simulink model "gm_uz_pmsm_model_6LUT_pd_vnl"  (R2023b)
settings: Solver=FixedStepAuto  StartTime=0.0  StopTime=0.05  RelTol=1e-3
PreLoadFcn:
  | uz_pmsm_model_init_parameter
PostLoadFcn:
  | % Import the data from Excel for a lookup table
  | FluxMapData = readtable('C:\Users\Philipp\ultrazohm\ultrazohm_sw\ip_cores\uz_pmsm_model\FluxMapData_2023-05-26_13-07-57.csv');
  | % Row indices for lookup table
  | d_current_in_d_axis = FluxMapData(8:27,1:end);
  | % Column indices for lookup table
  | q_current_in_d_axis = FluxMapData(29:48,1:end);
  | % Output values for lookup table
  | d_Flux_d_axis = FluxMapData(50:69,1:end);
undefined symbols (not defined in the file or in its folder): ad1, ad2, ad3, ad4, ad5, ad6, aq1, aq2, aq3, aq4, aq5, aq6, d_current_d_Flux, d_current_q_Flux, entkopplung_dynamic, entkopplung_linear, entkopplung_static, Fid1_Giq1, Fid2_Giq2, Flux_d, Flux_q, friction_coefficient, inertia, Ki_Bo_d, Ki_Bo_q, Kp_Bo_d, Kp_Bo_q, L_d, L_q, Ldq, parameter_nachfuerung, polepair, praediktion_entkopplung_nonlinear, psi_pm, q_current_d_Flux, q_current_q_Flux, R_1, simulate_mechanical, simulate_nonlinear_modell, simulate_open_loop, static_friction_torque, tau_sum, ts, ts_regler
libraries: hdlmdlgenlib x19, simulink x2, slpidlib x2
(part 4 of 4)

== system gm_uz_pmsm_model_6LUT_pd_vnl/uz_pmsm_model_6LUT/Product41 ==
  In1 : Inport
  In2 : Inport  Port=2
  Product41 : Product  Inputs=**  OutDataTypeStr=double  SampleTime=1e-08
  Product41_pd1 : Delay  DelayLength=6
  Out1 : Outport
  wires:
  Product41_pd1/1 -> Out1/1
  Product41/1 -> Product41_pd1/1
  In2/1 -> Product41/2
  In1/1 -> Product41/1

== system gm_uz_pmsm_model_6LUT_pd_vnl/uz_pmsm_model_6LUT/Product42 ==
  In1 : Inport
  In2 : Inport  Port=2
  Product42 : Product  Inputs=**  OutDataTypeStr=double  SampleTime=1e-08
  Product42_pd1 : Delay  DelayLength=6
  Out1 : Outport
  wires:
  Product42_pd1/1 -> Out1/1
  Product42/1 -> Product42_pd1/1
  In2/1 -> Product42/2
  In1/1 -> Product42/1

== system gm_uz_pmsm_model_6LUT_pd_vnl/uz_pmsm_model_6LUT/Product43 ==
  In1 : Inport
  In2 : Inport  Port=2
  Product43 : Product  Inputs=**  OutDataTypeStr=double  SampleTime=1e-08
  Product43_pd1 : Delay  DelayLength=6
  Out1 : Outport
  wires:
  Product43_pd1/1 -> Out1/1
  Product43/1 -> Product43_pd1/1
  In2/1 -> Product43/2
  In1/1 -> Product43/1

== system gm_uz_pmsm_model_6LUT_pd_vnl/uz_pmsm_model_6LUT/Product5 ==
  In1 : Inport
  In2 : Inport  Port=2
  Product5 : Product  Inputs=**  OutDataTypeStr=double  SampleTime=1e-08
  Product5_pd1 : Delay  DelayLength=6
  Out1 : Outport
  wires:
  Product5_pd1/1 -> Out1/1
  Product5/1 -> Product5_pd1/1
  In2/1 -> Product5/2
  In1/1 -> Product5/1

== system gm_uz_pmsm_model_6LUT_pd_vnl/uz_pmsm_model_6LUT/Product51 ==
  In1 : Inport
  In2 : Inport  Port=2
  Product51 : Product  Inputs=**  OutDataTypeStr=double  SampleTime=1e-08
  Product51_pd1 : Delay  DelayLength=6
  Out1 : Outport
  wires:
  Product51_pd1/1 -> Out1/1
  Product51/1 -> Product51_pd1/1
  In2/1 -> Product51/2
  In1/1 -> Product51/1

== system gm_uz_pmsm_model_6LUT_pd_vnl/uz_pmsm_model_6LUT/Product52 ==
  In1 : Inport
  In2 : Inport  Port=2
  Product52 : Product  Inputs=**  OutDataTypeStr=double  SampleTime=1e-08
  Product52_pd1 : Delay  DelayLength=6
  Out1 : Outport
  wires:
  Product52_pd1/1 -> Out1/1
  Product52/1 -> Product52_pd1/1
  In2/1 -> Product52/2
  In1/1 -> Product52/1

== system gm_uz_pmsm_model_6LUT_pd_vnl/uz_pmsm_model_6LUT/Product6 ==
  In1 : Inport
  In2 : Inport  Port=2
  Product6 : Product  Inputs=**  OutDataTypeStr=double  SampleTime=1e-08
  Product6_pd1 : Delay  DelayLength=6
  Out1 : Outport
  wires:
  Product6_pd1/1 -> Out1/1
  Product6/1 -> Product6_pd1/1
  In2/1 -> Product6/2
  In1/1 -> Product6/1

== system gm_uz_pmsm_model_6LUT_pd_vnl/uz_pmsm_model_6LUT/Product61 ==
  In1 : Inport
  In2 : Inport  Port=2
  Product61 : Product  Inputs=**  OutDataTypeStr=double  SampleTime=1e-08
  Product61_pd1 : Delay  DelayLength=6
  Out1 : Outport
  wires:
  Product61_pd1/1 -> Out1/1
  Product61/1 -> Product61_pd1/1
  In2/1 -> Product61/2
  In1/1 -> Product61/1

== system gm_uz_pmsm_model_6LUT_pd_vnl/uz_pmsm_model_6LUT/Product7 ==
  In1 : Inport
  In2 : Inport  Port=2
  Product7 : Product  Inputs=**  OutDataTypeStr=double  SampleTime=1e-08
  Product7_pd1 : Delay  DelayLength=6
  Out1 : Outport
  wires:
  Product7_pd1/1 -> Out1/1
  Product7/1 -> Product7_pd1/1
  In2/1 -> Product7/2
  In1/1 -> Product7/1

== system gm_uz_pmsm_model_6LUT_pd_vnl/uz_pmsm_model_6LUT/Product71 ==
  In1 : Inport
  In2 : Inport  Port=2
  Product71 : Product  Inputs=**  OutDataTypeStr=double  SampleTime=1e-08
  Product71_pd1 : Delay  DelayLength=6
  Out1 : Outport
  wires:
  Product71_pd1/1 -> Out1/1
  Product71/1 -> Product71_pd1/1
  In2/1 -> Product71/2
  In1/1 -> Product71/1

== system gm_uz_pmsm_model_6LUT_pd_vnl/uz_pmsm_model_6LUT/Product7_to_gain ==
  In1 : Inport
  Product7_to_gain : Gain  Gain=double(0.5)
  Product7_to_gain_pd1 : Delay  DelayLength=3
  Out1 : Outport
  wires:
  Product7_to_gain_pd1/1 -> Out1/1
  Product7_to_gain/1 -> Product7_to_gain_pd1/1
  In1/1 -> Product7_to_gain/1

== system gm_uz_pmsm_model_6LUT_pd_vnl/uz_pmsm_model_6LUT/Product8 ==
  In1 : Inport
  In2 : Inport  Port=2
  Product8 : Product  Inputs=**  OutDataTypeStr=double  SampleTime=1e-08
  Product8_pd1 : Delay  DelayLength=6
  Out1 : Outport
  wires:
  Product8_pd1/1 -> Out1/1
  Product8/1 -> Product8_pd1/1
  In2/1 -> Product8/2
  In1/1 -> Product8/1

== system gm_uz_pmsm_model_6LUT_pd_vnl/uz_pmsm_model_6LUT/Product81 ==
  In1 : Inport
  In2 : Inport  Port=2
  Product81 : Product  Inputs=*/  OutDataTypeStr=double  SampleTime=1e-08
  Product81_pd1 : Delay  DelayLength=31
  Out1 : Outport
  wires:
  Product81_pd1/1 -> Out1/1
  Product81/1 -> Product81_pd1/1
  In2/1 -> Product81/2
  In1/1 -> Product81/1

== system gm_uz_pmsm_model_6LUT_pd_vnl/uz_pmsm_model_6LUT/Product9 ==
  In1 : Inport
  In2 : Inport  Port=2
  Product9 : Product  Inputs=**  OutDataTypeStr=double  SampleTime=1e-08
  Product9_pd1 : Delay  DelayLength=6
  Out1 : Outport
  wires:
  Product9_pd1/1 -> Out1/1
  Product9/1 -> Product9_pd1/1
  In2/1 -> Product9/2
  In1/1 -> Product9/1

== system gm_uz_pmsm_model_6LUT_pd_vnl/uz_pmsm_model_6LUT/Product91 ==
  In1 : Inport
  In2 : Inport  Port=2
  Product91 : Product  Inputs=**  OutDataTypeStr=double  SampleTime=1e-08
  Product91_pd1 : Delay  DelayLength=6
  Out1 : Outport
  wires:
  Product91_pd1/1 -> Out1/1
  Product91/1 -> Product91_pd1/1
  In2/1 -> Product91/2
  In1/1 -> Product91/1

== system gm_uz_pmsm_model_6LUT_pd_vnl/uz_pmsm_model_6LUT/Product92 ==
  In1 : Inport
  In2 : Inport  Port=2
  Product92 : Product  Inputs=**  OutDataTypeStr=double  SampleTime=1e-08
  Product92_pd1 : Delay  DelayLength=6
  Out1 : Outport
  wires:
  Product92_pd1/1 -> Out1/1
  Product92/1 -> Product92_pd1/1
  In2/1 -> Product92/2
  In1/1 -> Product92/1

== system gm_uz_pmsm_model_6LUT_pd_vnl/uz_pmsm_model_6LUT/Product93 ==
  In1 : Inport
  In2 : Inport  Port=2
  Product93 : Product  Inputs=**  OutDataTypeStr=double  SampleTime=1e-08
  Product93_pd1 : Delay  DelayLength=6
  Out1 : Outport
  wires:
  Product93_pd1/1 -> Out1/1
  Product93/1 -> Product93_pd1/1
  In2/1 -> Product93/2
  In1/1 -> Product93/1

== system gm_uz_pmsm_model_6LUT_pd_vnl/uz_pmsm_model_6LUT/Product94 ==
  In1 : Inport
  In2 : Inport  Port=2
  Product94 : Product  Inputs=*/  OutDataTypeStr=double  SampleTime=1e-08
  Product94_pd1 : Delay  DelayLength=31
  Out1 : Outport
  wires:
  Product94_pd1/1 -> Out1/1
  Product94/1 -> Product94_pd1/1
  In2/1 -> Product94/2
  In1/1 -> Product94/1

== system gm_uz_pmsm_model_6LUT_pd_vnl/uz_pmsm_model_6LUT/Sign1 ==
  In1 : Inport
  Sign1 : Signum  SampleTime=1e-08
  Out1 : Outport
  wires:
  Sign1/1 -> Out1/1
  In1/1 -> Sign1/1

== system gm_uz_pmsm_model_6LUT_pd_vnl/uz_pmsm_model_6LUT/Sum ==
  In1 : Inport
  In2 : Inport  Port=2
  Sum : Sum  Inputs=+-  OutDataTypeStr=double  SampleTime=1e-08
  Sum_pd1 : Delay  DelayLength=6
  Out1 : Outport
  wires:
  Sum_pd1/1 -> Out1/1
  Sum/1 -> Sum_pd1/1
  In2/1 -> Sum/2
  In1/1 -> Sum/1

== system gm_uz_pmsm_model_6LUT_pd_vnl/uz_pmsm_model_6LUT/Sum1 ==
  In1 : Inport
  In2 : Inport  Port=2
  Sum1 : Sum  Inputs=+-  OutDataTypeStr=double  SampleTime=1e-08
  Sum1_pd1 : Delay  DelayLength=6
  Out1 : Outport
  wires:
  Sum1_pd1/1 -> Out1/1
  Sum1/1 -> Sum1_pd1/1
  In2/1 -> Sum1/2
  In1/1 -> Sum1/1

== system gm_uz_pmsm_model_6LUT_pd_vnl/uz_pmsm_model_6LUT/Sum10 ==
  In1 : Inport
  In2 : Inport  Port=2
  Sum10 : Sum  Inputs=+-  OutDataTypeStr=double  SampleTime=1e-08
  Sum10_pd1 : Delay  DelayLength=6
  Out1 : Outport
  wires:
  Sum10_pd1/1 -> Out1/1
  Sum10/1 -> Sum10_pd1/1
  In2/1 -> Sum10/2
  In1/1 -> Sum10/1

== system gm_uz_pmsm_model_6LUT_pd_vnl/uz_pmsm_model_6LUT/Sum101 ==
  In1 : Inport
  In2 : Inport  Port=2
  Sum101 : Sum  Inputs=+-  OutDataTypeStr=double  SampleTime=1e-08
  Sum101_pd1 : Delay  DelayLength=6
  Out1 : Outport
  wires:
  Sum101_pd1/1 -> Out1/1
  Sum101/1 -> Sum101_pd1/1
  In2/1 -> Sum101/2
  In1/1 -> Sum101/1

== system gm_uz_pmsm_model_6LUT_pd_vnl/uz_pmsm_model_6LUT/Sum11 ==
  In1 : Inport
  In2 : Inport  Port=2
  Sum11 : Sum  Inputs=+-  OutDataTypeStr=double  SampleTime=1e-08
  Sum11_pd1 : Delay  DelayLength=6
  Out1 : Outport
  wires:
  Sum11_pd1/1 -> Out1/1
  Sum11/1 -> Sum11_pd1/1
  In2/1 -> Sum11/2
  In1/1 -> Sum11/1

== system gm_uz_pmsm_model_6LUT_pd_vnl/uz_pmsm_model_6LUT/Sum12 ==
  In1 : Inport
  In2 : Inport  Port=2
  Sum12 : Sum  OutDataTypeStr=double  SampleTime=1e-08
  Sum12_pd1 : Delay  DelayLength=6
  Out1 : Outport
  wires:
  Sum12_pd1/1 -> Out1/1
  Sum12/1 -> Sum12_pd1/1
  In2/1 -> Sum12/2
  In1/1 -> Sum12/1

== system gm_uz_pmsm_model_6LUT_pd_vnl/uz_pmsm_model_6LUT/Sum13 ==
  In1 : Inport
  In2 : Inport  Port=2
  Sum13 : Sum  OutDataTypeStr=double  SampleTime=1e-08
  Sum13_pd1 : Delay  DelayLength=6
  Out1 : Outport
  wires:
  Sum13_pd1/1 -> Out1/1
  Sum13/1 -> Sum13_pd1/1
  In2/1 -> Sum13/2
  In1/1 -> Sum13/1

== system gm_uz_pmsm_model_6LUT_pd_vnl/uz_pmsm_model_6LUT/Sum14 ==
  In1 : Inport
  In2 : Inport  Port=2
  Sum14 : Sum  Inputs=+-  OutDataTypeStr=double  SampleTime=1e-08
  Sum14_pd1 : Delay  DelayLength=6
  Out1 : Outport
  wires:
  Sum14_pd1/1 -> Out1/1
  Sum14/1 -> Sum14_pd1/1
  In2/1 -> Sum14/2
  In1/1 -> Sum14/1

== system gm_uz_pmsm_model_6LUT_pd_vnl/uz_pmsm_model_6LUT/Sum2 ==
  In1 : Inport
  In2 : Inport  Port=2
  Sum2 : Sum  Inputs=+-  OutDataTypeStr=double  SampleTime=1e-08
  Sum2_pd1 : Delay  DelayLength=6
  Out1 : Outport
  wires:
  Sum2_pd1/1 -> Out1/1
  Sum2/1 -> Sum2_pd1/1
  In2/1 -> Sum2/2
  In1/1 -> Sum2/1

== system gm_uz_pmsm_model_6LUT_pd_vnl/uz_pmsm_model_6LUT/Sum21 ==
  In1 : Inport
  In2 : Inport  Port=2
  Sum21 : Sum  Inputs=+-  OutDataTypeStr=double  SampleTime=1e-08
  Sum21_pd1 : Delay  DelayLength=6
  Out1 : Outport
  wires:
  Sum21_pd1/1 -> Out1/1
  Sum21/1 -> Sum21_pd1/1
  In2/1 -> Sum21/2
  In1/1 -> Sum21/1

== system gm_uz_pmsm_model_6LUT_pd_vnl/uz_pmsm_model_6LUT/Sum22 ==
  In1 : Inport
  In2 : Inport  Port=2
  Sum22 : Sum  Inputs=+-  OutDataTypeStr=double  SampleTime=1e-08
  Sum22_pd1 : Delay  DelayLength=6
  Out1 : Outport
  wires:
  Sum22_pd1/1 -> Out1/1
  Sum22/1 -> Sum22_pd1/1
  In2/1 -> Sum22/2
  In1/1 -> Sum22/1

== system gm_uz_pmsm_model_6LUT_pd_vnl/uz_pmsm_model_6LUT/Sum23 ==
  In1 : Inport
  In2 : Inport  Port=2
  Sum23 : Sum  Inputs=+-  OutDataTypeStr=double  SampleTime=1e-08
  Sum23_pd1 : Delay  DelayLength=6
  Out1 : Outport
  wires:
  Sum23_pd1/1 -> Out1/1
  Sum23/1 -> Sum23_pd1/1
  In2/1 -> Sum23/2
  In1/1 -> Sum23/1

== system gm_uz_pmsm_model_6LUT_pd_vnl/uz_pmsm_model_6LUT/Sum24 ==
  In1 : Inport
  In2 : Inport  Port=2
  Sum24 : Sum  Inputs=+-  OutDataTypeStr=double  SampleTime=1e-08
  Sum24_pd1 : Delay  DelayLength=6
  Out1 : Outport
  wires:
  Sum24_pd1/1 -> Out1/1
  Sum24/1 -> Sum24_pd1/1
  In2/1 -> Sum24/2
  In1/1 -> Sum24/1

== system gm_uz_pmsm_model_6LUT_pd_vnl/uz_pmsm_model_6LUT/Sum3 ==
  In1 : Inport
  In2 : Inport  Port=2
  Sum3 : Sum  Inputs=+-  OutDataTypeStr=double  SampleTime=1e-08
  Sum3_pd1 : Delay  DelayLength=6
  Out1 : Outport
  wires:
  Sum3_pd1/1 -> Out1/1
  Sum3/1 -> Sum3_pd1/1
  In2/1 -> Sum3/2
  In1/1 -> Sum3/1

== system gm_uz_pmsm_model_6LUT_pd_vnl/uz_pmsm_model_6LUT/Sum31 ==
  In1 : Inport
  In2 : Inport  Port=2
  Sum31 : Sum  OutDataTypeStr=double  SampleTime=1e-08
  Sum31_pd1 : Delay  DelayLength=6
  Out1 : Outport
  wires:
  Sum31_pd1/1 -> Out1/1
  Sum31/1 -> Sum31_pd1/1
  In2/1 -> Sum31/2
  In1/1 -> Sum31/1

== system gm_uz_pmsm_model_6LUT_pd_vnl/uz_pmsm_model_6LUT/Sum32 ==
  In1 : Inport
  In2 : Inport  Port=2
  Sum32 : Sum  Inputs=+-  OutDataTypeStr=double  SampleTime=1e-08
  Sum32_pd1 : Delay  DelayLength=6
  Out1 : Outport
  wires:
  Sum32_pd1/1 -> Out1/1
  Sum32/1 -> Sum32_pd1/1
  In2/1 -> Sum32/2
  In1/1 -> Sum32/1

== system gm_uz_pmsm_model_6LUT_pd_vnl/uz_pmsm_model_6LUT/Sum3_stage2 ==
  In1 : Inport
  In2 : Inport  Port=2
  Sum3_stage2 : Sum  OutDataTypeStr=double  SampleTime=1e-08
  Sum3_stage2_pd1 : Delay  DelayLength=6
  Out1 : Outport
  wires:
  Sum3_stage2_pd1/1 -> Out1/1
  Sum3_stage2/1 -> Sum3_stage2_pd1/1
  In2/1 -> Sum3_stage2/2
  In1/1 -> Sum3_stage2/1

== system gm_uz_pmsm_model_6LUT_pd_vnl/uz_pmsm_model_6LUT/Sum3_stage21 ==
  In1 : Inport
  In2 : Inport  Port=2
  Sum3_stage21 : Sum  Inputs=+-  OutDataTypeStr=double  SampleTime=1e-08
  Sum3_stage21_pd1 : Delay  DelayLength=6
  Out1 : Outport
  wires:
  Sum3_stage21_pd1/1 -> Out1/1
  Sum3_stage21/1 -> Sum3_stage21_pd1/1
  In2/1 -> Sum3_stage21/2
  In1/1 -> Sum3_stage21/1

== system gm_uz_pmsm_model_6LUT_pd_vnl/uz_pmsm_model_6LUT/Sum3_stage3 ==
  In1 : Inport
  In2 : Inport  Port=2
  Sum3_stage3 : Sum  Inputs=+-  OutDataTypeStr=double  SampleTime=1e-08
  Sum3_stage3_pd1 : Delay  DelayLength=6
  Out1 : Outport
  wires:
  Sum3_stage3_pd1/1 -> Out1/1
  Sum3_stage3/1 -> Sum3_stage3_pd1/1
  In2/1 -> Sum3_stage3/2
  In1/1 -> Sum3_stage3/1

== system gm_uz_pmsm_model_6LUT_pd_vnl/uz_pmsm_model_6LUT/Sum3_stage31 ==
  In1 : Inport
  In2 : Inport  Port=2
  Sum3_stage31 : Sum  Inputs=+-  OutDataTypeStr=double  SampleTime=1e-08
  Sum3_stage31_pd1 : Delay  DelayLength=6
  Out1 : Outport
  wires:
  Sum3_stage31_pd1/1 -> Out1/1
  Sum3_stage31/1 -> Sum3_stage31_pd1/1
  In2/1 -> Sum3_stage31/2
  In1/1 -> Sum3_stage31/1

== system gm_uz_pmsm_model_6LUT_pd_vnl/uz_pmsm_model_6LUT/Sum3_stage4 ==
  In1 : Inport
  In2 : Inport  Port=2
  Sum3_stage4 : Sum  OutDataTypeStr=double  SampleTime=1e-08
  Sum3_stage4_pd1 : Delay  DelayLength=6
  Out1 : Outport
  wires:
  Sum3_stage4_pd1/1 -> Out1/1
  Sum3_stage4/1 -> Sum3_stage4_pd1/1
  In2/1 -> Sum3_stage4/2
  In1/1 -> Sum3_stage4/1

== system gm_uz_pmsm_model_6LUT_pd_vnl/uz_pmsm_model_6LUT/Sum4 ==
  In1 : Inport
  In2 : Inport  Port=2
  Sum4 : Sum  Inputs=+-  OutDataTypeStr=double  SampleTime=1e-08
  Sum4_pd1 : Delay  DelayLength=6
  Out1 : Outport
  wires:
  Sum4_pd1/1 -> Out1/1
  Sum4/1 -> Sum4_pd1/1
  In2/1 -> Sum4/2
  In1/1 -> Sum4/1

== system gm_uz_pmsm_model_6LUT_pd_vnl/uz_pmsm_model_6LUT/Sum41 ==
  In1 : Inport
  In2 : Inport  Port=2
  Sum41 : Sum  OutDataTypeStr=double  SampleTime=1e-08
  Sum41_pd1 : Delay  DelayLength=6
  Out1 : Outport
  wires:
  Sum41_pd1/1 -> Out1/1
  Sum41/1 -> Sum41_pd1/1
  In2/1 -> Sum41/2
  In1/1 -> Sum41/1

== system gm_uz_pmsm_model_6LUT_pd_vnl/uz_pmsm_model_6LUT/Sum42 ==
  In1 : Inport
  In2 : Inport  Port=2
  Sum42 : Sum  OutDataTypeStr=double  SampleTime=1e-08
  Sum42_pd1 : Delay  DelayLength=6
  Out1 : Outport
  wires:
  Sum42_pd1/1 -> Out1/1
  Sum42/1 -> Sum42_pd1/1
  In2/1 -> Sum42/2
  In1/1 -> Sum42/1

== system gm_uz_pmsm_model_6LUT_pd_vnl/uz_pmsm_model_6LUT/Sum4_stage2 ==
  In1 : Inport
  In2 : Inport  Port=2
  Sum4_stage2 : Sum  Inputs=+-  OutDataTypeStr=double  SampleTime=1e-08
  Sum4_stage2_pd1 : Delay  DelayLength=6
  Out1 : Outport
  wires:
  Sum4_stage2_pd1/1 -> Out1/1
  Sum4_stage2/1 -> Sum4_stage2_pd1/1
  In2/1 -> Sum4_stage2/2
  In1/1 -> Sum4_stage2/1

== system gm_uz_pmsm_model_6LUT_pd_vnl/uz_pmsm_model_6LUT/Sum4_stage3 ==
  In1 : Inport
  In2 : Inport  Port=2
  Sum4_stage3 : Sum  Inputs=+-  OutDataTypeStr=double  SampleTime=1e-08
  Sum4_stage3_pd1 : Delay  DelayLength=6
  Out1 : Outport
  wires:
  Sum4_stage3_pd1/1 -> Out1/1
  Sum4_stage3/1 -> Sum4_stage3_pd1/1
  In2/1 -> Sum4_stage3/2
  In1/1 -> Sum4_stage3/1

== system gm_uz_pmsm_model_6LUT_pd_vnl/uz_pmsm_model_6LUT/Sum4_stage4 ==
  In1 : Inport
  In2 : Inport  Port=2
  Sum4_stage4 : Sum  Inputs=+-  OutDataTypeStr=double  SampleTime=1e-08
  Sum4_stage4_pd1 : Delay  DelayLength=6
  Out1 : Outport
  wires:
  Sum4_stage4_pd1/1 -> Out1/1
  Sum4_stage4/1 -> Sum4_stage4_pd1/1
  In2/1 -> Sum4_stage4/2
  In1/1 -> Sum4_stage4/1

== system gm_uz_pmsm_model_6LUT_pd_vnl/uz_pmsm_model_6LUT/Sum5 ==
  In1 : Inport
  In2 : Inport  Port=2
  Sum5 : Sum  Inputs=+-  OutDataTypeStr=double  SampleTime=1e-08
  Sum5_pd1 : Delay  DelayLength=6
  Out1 : Outport
  wires:
  Sum5_pd1/1 -> Out1/1
  Sum5/1 -> Sum5_pd1/1
  In2/1 -> Sum5/2
  In1/1 -> Sum5/1

== system gm_uz_pmsm_model_6LUT_pd_vnl/uz_pmsm_model_6LUT/Sum51 ==
  In1 : Inport
  In2 : Inport  Port=2
  Sum51 : Sum  OutDataTypeStr=double  SampleTime=1e-08
  Sum51_pd1 : Delay  DelayLength=6
  Out1 : Outport
  wires:
  Sum51_pd1/1 -> Out1/1
  Sum51/1 -> Sum51_pd1/1
  In2/1 -> Sum51/2
  In1/1 -> Sum51/1

== system gm_uz_pmsm_model_6LUT_pd_vnl/uz_pmsm_model_6LUT/Sum52 ==
  In1 : Inport
  In2 : Inport  Port=2
  Sum52 : Sum  OutDataTypeStr=double  SampleTime=1e-08
  Sum52_pd1 : Delay  DelayLength=6
  Out1 : Outport
  wires:
  Sum52_pd1/1 -> Out1/1
  Sum52/1 -> Sum52_pd1/1
  In2/1 -> Sum52/2
  In1/1 -> Sum52/1

== system gm_uz_pmsm_model_6LUT_pd_vnl/uz_pmsm_model_6LUT/Sum53 ==
  In1 : Inport
  In2 : Inport  Port=2
  Sum53 : Sum  OutDataTypeStr=double  SampleTime=1e-08
  Sum53_pd1 : Delay  DelayLength=6
  Out1 : Outport
  wires:
  Sum53_pd1/1 -> Out1/1
  Sum53/1 -> Sum53_pd1/1
  In2/1 -> Sum53/2
  In1/1 -> Sum53/1

== system gm_uz_pmsm_model_6LUT_pd_vnl/uz_pmsm_model_6LUT/Sum6 ==
  In1 : Inport
  In2 : Inport  Port=2
  Sum6 : Sum  Inputs=+-  OutDataTypeStr=double  SampleTime=1e-08
  Sum6_pd1 : Delay  DelayLength=6
  Out1 : Outport
  wires:
  Sum6_pd1/1 -> Out1/1
  Sum6/1 -> Sum6_pd1/1
  In2/1 -> Sum6/2
  In1/1 -> Sum6/1

== system gm_uz_pmsm_model_6LUT_pd_vnl/uz_pmsm_model_6LUT/Sum7 ==
  In1 : Inport
  In2 : Inport  Port=2
  Sum7 : Sum  Inputs=+-  OutDataTypeStr=double  SampleTime=1e-08
  Sum7_pd1 : Delay  DelayLength=6
  Out1 : Outport
  wires:
  Sum7_pd1/1 -> Out1/1
  Sum7/1 -> Sum7_pd1/1
  In2/1 -> Sum7/2
  In1/1 -> Sum7/1

== system gm_uz_pmsm_model_6LUT_pd_vnl/uz_pmsm_model_6LUT/Sum71 ==
  In1 : Inport
  In2 : Inport  Port=2
  Sum71 : Sum  Inputs=+-  OutDataTypeStr=double  SampleTime=1e-08
  Sum71_pd1 : Delay  DelayLength=6
  Out1 : Outport
  wires:
  Sum71_pd1/1 -> Out1/1
  Sum71/1 -> Sum71_pd1/1
  In2/1 -> Sum71/2
  In1/1 -> Sum71/1

== system gm_uz_pmsm_model_6LUT_pd_vnl/uz_pmsm_model_6LUT/Sum8 ==
  In1 : Inport
  In2 : Inport  Port=2
  Sum8 : Sum  OutDataTypeStr=double  SampleTime=1e-08
  Sum8_pd1 : Delay  DelayLength=6
  Out1 : Outport
  wires:
  Sum8_pd1/1 -> Out1/1
  Sum8/1 -> Sum8_pd1/1
  In2/1 -> Sum8/2
  In1/1 -> Sum8/1

== system gm_uz_pmsm_model_6LUT_pd_vnl/uz_pmsm_model_6LUT/Sum9 ==
  In1 : Inport
  In2 : Inport  Port=2
  Sum9 : Sum  Inputs=+-  OutDataTypeStr=double  SampleTime=1e-08
  Sum9_pd1 : Delay  DelayLength=6
  Out1 : Outport
  wires:
  Sum9_pd1/1 -> Out1/1
  Sum9/1 -> Sum9_pd1/1
  In2/1 -> Sum9/2
  In1/1 -> Sum9/1

== system gm_uz_pmsm_model_6LUT_pd_vnl/uz_pmsm_model_6LUT/Tanh ==
  In1 : Inport
  Tanh : Trigonometry  Operator=tanh  SampleTime=1e-08
  Tanh_pd1 : Delay  DelayLength=25
  Out1 : Outport
  wires:
  Tanh_pd1/1 -> Out1/1
  Tanh/1 -> Tanh_pd1/1
  In1/1 -> Tanh/1

== system gm_uz_pmsm_model_6LUT_pd_vnl/uz_pmsm_model_6LUT/Tanh1 ==
  In1 : Inport
  Tanh1 : Trigonometry  Operator=tanh  SampleTime=1e-08
  Tanh1_pd1 : Delay  DelayLength=25
  Out1 : Outport
  wires:
  Tanh1_pd1/1 -> Out1/1
  Tanh1/1 -> Tanh1_pd1/1
  In1/1 -> Tanh1/1

== system gm_uz_pmsm_model_6LUT_pd_vnl/uz_pmsm_model_6LUT/Tanh11 ==
  In1 : Inport
  Tanh11 : Trigonometry  Operator=cosh  SampleTime=1e-08
  Tanh11_pd1 : Delay  DelayLength=17
  Out1 : Outport
  wires:
  Tanh11_pd1/1 -> Out1/1
  Tanh11/1 -> Tanh11_pd1/1
  In1/1 -> Tanh11/1

== system gm_uz_pmsm_model_6LUT_pd_vnl/uz_pmsm_model_6LUT/Tanh12 ==
  In1 : Inport
  Tanh12 : Trigonometry  Operator=cosh  SampleTime=1e-08
  Tanh12_pd1 : Delay  DelayLength=17
  Out1 : Outport
  wires:
  Tanh12_pd1/1 -> Out1/1
  Tanh12/1 -> Tanh12_pd1/1
  In1/1 -> Tanh12/1

== system gm_uz_pmsm_model_6LUT_pd_vnl/uz_pmsm_model_6LUT/Tanh13 ==
  In1 : Inport
  Tanh13 : Trigonometry  Operator=tanh  SampleTime=1e-08
  Tanh13_pd1 : Delay  DelayLength=25
  Out1 : Outport
  wires:
  Tanh13_pd1/1 -> Out1/1
  Tanh13/1 -> Tanh13_pd1/1
  In1/1 -> Tanh13/1

== system gm_uz_pmsm_model_6LUT_pd_vnl/uz_pmsm_model_6LUT/Tanh2 ==
  In1 : Inport
  Tanh2 : Trigonometry  Operator=cosh  SampleTime=1e-08
  Tanh2_pd1 : Delay  DelayLength=17
  Out1 : Outport
  wires:
  Tanh2_pd1/1 -> Out1/1
  Tanh2/1 -> Tanh2_pd1/1
  In1/1 -> Tanh2/1

== system gm_uz_pmsm_model_6LUT_pd_vnl/uz_pmsm_model_6LUT/Tanh21 ==
  In1 : Inport
  Tanh21 : Trigonometry  Operator=cosh  SampleTime=1e-08
  Tanh21_pd1 : Delay  DelayLength=17
  Out1 : Outport
  wires:
  Tanh21_pd1/1 -> Out1/1
  Tanh21/1 -> Tanh21_pd1/1
  In1/1 -> Tanh21/1

== system gm_uz_pmsm_model_6LUT_pd_vnl/uz_pmsm_model_6LUT/Tanh3 ==
  In1 : Inport
  Tanh3 : Trigonometry  Operator=cosh  SampleTime=1e-08
  Tanh3_pd1 : Delay  DelayLength=17
  Out1 : Outport
  wires:
  Tanh3_pd1/1 -> Out1/1
  Tanh3/1 -> Tanh3_pd1/1
  In1/1 -> Tanh3/1

== system gm_uz_pmsm_model_6LUT_pd_vnl/uz_pmsm_model_6LUT/Tanh31 ==
  In1 : Inport
  Tanh31 : Trigonometry  Operator=cosh  SampleTime=1e-08
  Tanh31_pd1 : Delay  DelayLength=17
  Out1 : Outport
  wires:
  Tanh31_pd1/1 -> Out1/1
  Tanh31/1 -> Tanh31_pd1/1
  In1/1 -> Tanh31/1

== system gm_uz_pmsm_model_6LUT_pd_vnl/uz_pmsm_model_6LUT/Tanh4 ==
  In1 : Inport
  Tanh4 : Trigonometry  Operator=cosh  SampleTime=1e-08
  Tanh4_pd1 : Delay  DelayLength=17
  Out1 : Outport
  wires:
  Tanh4_pd1/1 -> Out1/1
  Tanh4/1 -> Tanh4_pd1/1
  In1/1 -> Tanh4/1

== system gm_uz_pmsm_model_6LUT_pd_vnl/uz_pmsm_model_6LUT/Tanh41 ==
  In1 : Inport
  Tanh41 : Trigonometry  Operator=cosh  SampleTime=1e-08
  Tanh41_pd1 : Delay  DelayLength=17
  Out1 : Outport
  wires:
  Tanh41_pd1/1 -> Out1/1
  Tanh41/1 -> Tanh41_pd1/1
  In1/1 -> Tanh41/1

== system gm_uz_pmsm_model_6LUT_pd_vnl/uz_pmsm_model_6LUT/Tanh5 ==
  In1 : Inport
  Tanh5 : Trigonometry  Operator=tanh  SampleTime=1e-08
  Tanh5_pd1 : Delay  DelayLength=25
  Out1 : Outport
  wires:
  Tanh5_pd1/1 -> Out1/1
  Tanh5/1 -> Tanh5_pd1/1
  In1/1 -> Tanh5/1

== system gm_uz_pmsm_model_6LUT_pd_vnl/uz_pmsm_model_6LUT_vnl/mechanical_system ==
  note: This delay breaks the algebraic loop between mechanical and electrical system.
      | Introduces a delay of 500ns.
  reset : Inport
  M_Mi : Inport  Port=2
  mu : Inport  Port=3
  M_n0 : Inport  Port=4
  reciprocal_J : Inport  Port=5
  load_torque : Inport  Port=6
  Abs : Abs  SaturateOnIntegerOverflow=off
  Delay : Delay  DelayLength=1
  Product11 : Product
  Product12 : Product
  Product4 : Product
  Sign1 : Signum
  Sum : Sum  Inputs=|+-  OutDataTypeStr=double
  Sum1 : Sum  Inputs=|+-
  Sum5 : Sum  Inputs=|++
  integrator1 : Subsystem
  omega_mech : Outport
  wires:
  Delay/1 -> Sum1/1
  Product4/1 -> Sum/2
  Sum/1 -> Delay/1
  load_torque/1 -> Sum1/2
  Sum1/1 -> Product11/2
  M_Mi/1 -> Sum/1
  reciprocal_J/1 -> Product11/1
  M_n0/1 -> Sum5/2
  mu/1 -> Product12/1
  Product12/1 -> Sum5/1
  reset/1 -> integrator1/1(reset)
  Abs/1 -> Product12/2
  integrator1/1(outt) -> omega_mech/1, Abs/1, Sign1/1
  Sign1/1 -> Product4/2
  Sum5/1 -> Product4/1
  Product11/1 -> integrator1/2(in)

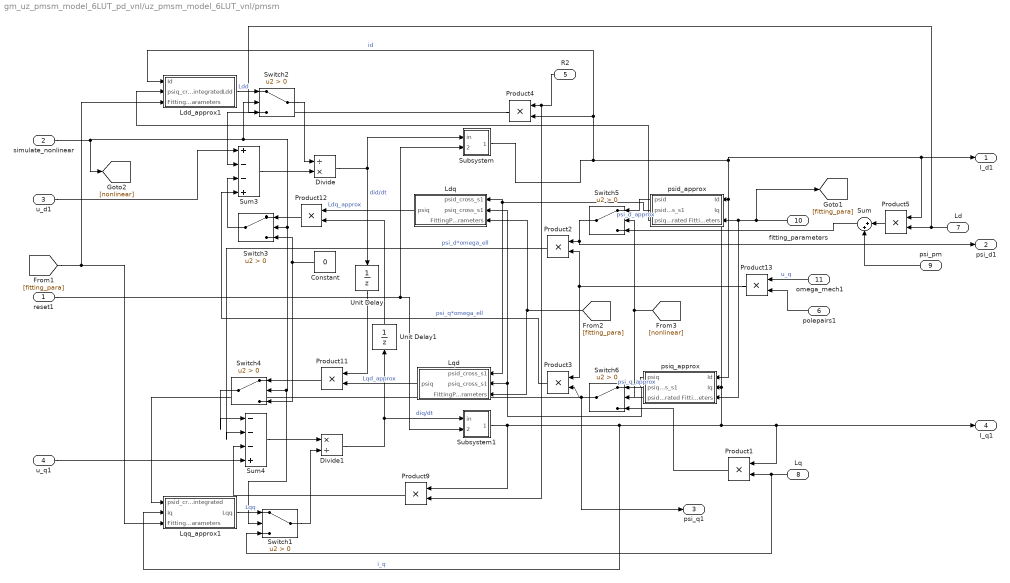
== system gm_uz_pmsm_model_6LUT_pd_vnl/uz_pmsm_model_6LUT_vnl/pmsm ==
  reset1 : Inport
  simulate_nonlinear : Inport  Port=2
  u_d1 : Inport  Port=3
  u_q1 : Inport  Port=4
  R2 : Inport  Port=5
  polepairs1 : Inport  Port=6
  Ld : Inport  Port=7
  Lq : Inport  Port=8
  psi_pm : Inport  Port=9
  fitting_parameters : Inport  Port=10
  omega_mech1 : Inport  Port=11
  Constant : Constant  Value=0  SampleTime=ts
  Divide : Product  Inputs=/*
  Divide1 : Product  Inputs=*/  OutDataTypeStr=Inherit: Same as first input
  Ldd_approx1 : Subsystem
  Ldq : Subsystem
  Lqd : Subsystem
  Lqq_approx1 : Subsystem
  Product{1,3..5,12..13} (6 alike) : Product
  Product11 : Product  OutDataTypeStr=double
  Product2 : Product  OutDataTypeStr=double
  Product9 : Product  OutDataTypeStr=Inherit: Same as first input
  Subsystem : Subsystem
  Subsystem1 : Subsystem
  Sum : Sum  Inputs=|++
  Sum3 : Sum  Inputs=|+--+
  Sum4 : Sum  Inputs=|---+
  Switch{1..6} (6 alike) : Switch  Criteria=u2 > Threshold  SaturateOnIntegerOverflow=off  InputSameDT=off
  Unit Delay : UnitDelay  SampleTime=-1  HasFrameUpgradeWarning=on
  Unit Delay1 : UnitDelay  SampleTime=-1  HasFrameUpgradeWarning=on
  psid_approx : Subsystem
  psiq_approx : Subsystem
  I_d1 : Outport
  psi_d1 : Outport  Port=2
  psi_q1 : Outport  Port=3
  I_q1 : Outport  Port=4
  wires:
  psid_approx/3(psiq_cross_s1_integrated) -> Ldd_approx1/2(psiq_cross_s1_integrated)
  psiq_approx/3(psid_cross_s1_integrated) -> Lqq_approx1/1(psid_cross_s1_integrated)
  psid_approx/2(psid_cross_s1) -> Lqd/1(psid_cross_s1), Ldq/1(psid_cross_s1)
  psiq_approx/2(psiq_cross_s1) -> Lqd/2(psiq_cross_s1), Ldq/2(psiq_cross_s1)
  [fitting_para] -> Lqd/3(FittingParameters), Ldq/3(FittingParameters)
  [fitting_para] -> Lqq_approx1/3(FittingParameters), Ldd_approx1/3(FittingParameters)
  Product1/1 -> Switch6/3
  Lq/1 -> Product1/2, Switch1/3
  [nonlinear] -> Switch6/2, Switch5/2
  Switch6/1 -> Product3/2, psi_q1/1
  psiq_approx/1(psiq) -> Switch6/1  "psi_q_approx"
  Sum/1 -> Switch5/3
  psi_pm/1 -> Sum/2
  Ld/1 -> Product5/2, Switch2/3
  Product5/1 -> Sum/1
  Switch5/1 -> Product2/1, psi_d1/1
  psid_approx/1(psid) -> Switch5/1  "psi_d_approx"
  simulate_nonlinear/1 -> [nonlinear], Switch2/2, Switch3/2, Switch4/2, Switch1/2
  Switch4/1 -> Sum4/1
  Product11/1 -> Switch4/1
  Constant/1 -> Switch3/3, Switch4/3
  Switch3/1 -> Sum3/3
  Product12/1 -> Switch3/1
  Switch2/1 -> Divide/1
  Ldd_approx1/1(Ldd) -> Switch2/1  "Ldd"
  Switch1/1 -> Divide1/2
  Lqq_approx1/1(Lqq) -> Switch1/1  "Lqq"
  fitting_parameters/1 -> psid_approx/3(FittingParameters), psiq_approx/3(FittingParameters), [fitting_para]
  omega_mech1/1 -> Product13/1  "u_q"
  Ldq/1(psiq) -> Product12/1  "Ldq_approx"
  Lqd/1(psiq) -> Product11/2  "Lqd_approx"
  Unit Delay1/1 -> Product12/2
  Unit Delay/1 -> Product11/1
  Product2/1 -> Sum4/2  "psi_d*omega_ell"
  Product4/1 -> Sum3/2
  Product3/1 -> Sum3/4  "psi_q*omega_ell"
  Subsystem1/1(outt) -> Product9/1, psiq_approx/2(Iq), psid_approx/2(Iq), Product1/1, I_q1/1, Lqq_approx1/2(Iq)  "i_q"
  Subsystem/1(outt) -> psiq_approx/1(Id), psid_approx/1(Id), I_d1/1, Product5/1, Product4/2, Ldd_approx1/1(Id)  "id"
  R2/1 -> Product4/1, Product9/2
  u_d1/1 -> Sum3/1
  reset1/1 -> Subsystem1/2(reset), Subsystem/2(reset)
  Product9/1 -> Sum4/3
  Sum3/1 -> Divide/2
  Divide/1 -> Subsystem/1(in), Unit Delay/1  "did/dt"
  Product13/1 -> Product2/2, Product3/1
  polepairs1/1 -> Product13/2
  Divide1/1 -> Subsystem1/1(in), Unit Delay1/1  "diq/dt"
  u_q1/1 -> Sum4/4
  Sum4/1 -> Divide1/1

== system gm_uz_pmsm_model_6LUT_pd_vnl/uz_pmsm_model_6LUT_vnl/torque_calculation ==
  I_d : Inport
  psi_d : Inport  Port=2
  psi_q : Inport  Port=3
  polepairs : Inport  Port=4
  I_q : Inport  Port=5
  Factor : Gain  Gain=(3/2)
  Product2 : Product
  Product3 : Product
  Product9 : Product
  Sum3 : Sum  Inputs=-|+
  M_Mi : Outport
  wires:
  Factor/1 -> Product9/1  "M_Mi"
  polepairs/1 -> Product9/2
  Product9/1 -> M_Mi/1  "M_Mi"
  I_q/1 -> Product3/2
  I_d/1 -> Product2/1
  psi_d/1 -> Product3/1
  psi_q/1 -> Product2/2
  Product2/1 -> Sum3/1
  Product3/1 -> Sum3/2
  Sum3/1 -> Factor/1

== system gm_uz_pmsm_model_6LUT_pd_vnl/Compare/Assert_outputs/RelErrCheck ==
  In1 : Inport
  In2 : Inport  Port=2
  "RelativeErrorCheck " : MATLAB Function  TreatAsAtomicUnit=on
  Out1 : Outport  VectorParamsAs1DForOutWhenUnconnected=off
  wires:
  "RelativeErrorCheck "/1(y) -> Out1/1
  In1/1 -> "RelativeErrorCheck "/1(P)
  In2/1 -> "RelativeErrorCheck "/2(R)

== system gm_uz_pmsm_model_6LUT_pd_vnl/Current_Controller/Entkopplungen/Lineare_Entkopplung ==
  i_d : Inport
  i_q : Inport  Port=2
  omega_m : Inport  Port=3
  Constant1 : Constant  Value=psi_pm  SampleTime=-1
  Gain : Gain  Gain=L_q
  Gain1 : Gain  Gain=L_d
  Gain2 : Gain  Gain=polepair
  Product : Product
  Product1 : Product
  Sum6 : Sum  Inputs=|++
  u_d : Outport
  u_q : Outport  Port=2
  wires:
  omega_m/1 -> Gain2/1
  Sum6/1 -> Product1/1
  Product/1 -> u_d/1
  i_d/1 -> Gain1/1
  Constant1/1 -> Sum6/2
  i_q/1 -> Gain/1
  Product1/1 -> u_q/1
  Gain1/1 -> Sum6/1
  Gain2/1 -> Product1/2, Product/2
  Gain/1 -> Product/1

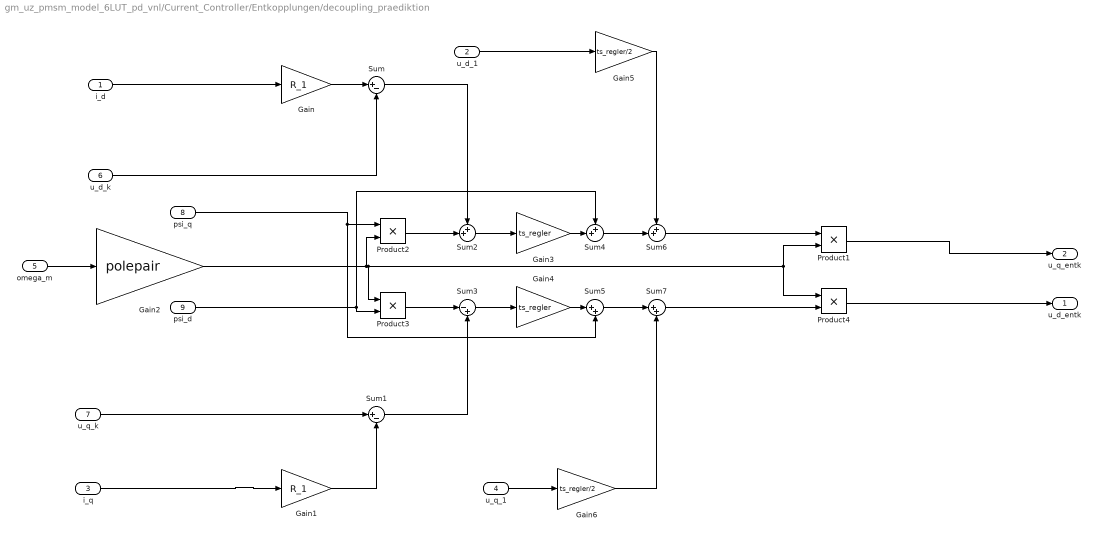
== system gm_uz_pmsm_model_6LUT_pd_vnl/Current_Controller/Entkopplungen/decoupling_praediktion ==
  i_d : Inport
  u_d_1 : Inport  Port=2
  i_q : Inport  Port=3
  u_q_1 : Inport  Port=4
  omega_m : Inport  Port=5
  u_d_k : Inport  Port=6
  u_q_k : Inport  Port=7
  psi_q : Inport  Port=8
  psi_d : Inport  Port=9
  Gain : Gain  Gain=R_1
  Gain1 : Gain  Gain=R_1
  Gain2 : Gain  Gain=polepair
  Gain3 : Gain  Gain=ts_regler
  Gain4 : Gain  Gain=ts_regler
  Gain5 : Gain  Gain=ts_regler/2
  Gain6 : Gain  Gain=ts_regler/2
  Product{1..4} (4 alike) : Product
  Sum : Sum  Inputs=|+-
  Sum1 : Sum  Inputs=|+-
  Sum2 : Sum  Inputs=++|
  Sum3 : Sum  Inputs=|-+
  Sum4 : Sum  Inputs=++|
  Sum5 : Sum  Inputs=|++
  Sum6 : Sum  Inputs=++|
  Sum7 : Sum  Inputs=|++
  u_d_entk : Outport
  u_q_entk : Outport  Port=2
  wires:
  psi_q/1 -> Sum5/2, Product2/1
  psi_d/1 -> Product3/2, Sum4/1
  Gain2/1 -> Product1/2, Product4/1, Product3/1, Product2/2
  u_d_k/1 -> Sum/2
  Gain/1 -> Sum/1
  u_q_k/1 -> Sum1/1
  Gain1/1 -> Sum1/2
  Product3/1 -> Sum3/1
  Product2/1 -> Sum2/2
  Sum/1 -> Sum2/1
  Sum1/1 -> Sum3/2
  Sum3/1 -> Gain4/1
  Sum2/1 -> Gain3/1
  Gain3/1 -> Sum4/2
  Gain4/1 -> Sum5/1
  u_d_1/1 -> Gain5/1
  Sum4/1 -> Sum6/2
  u_q_1/1 -> Gain6/1
  Gain5/1 -> Sum6/1
  Sum5/1 -> Sum7/1
  Gain6/1 -> Sum7/2
  Sum6/1 -> Product1/1
  Sum7/1 -> Product4/2
  omega_m/1 -> Gain2/1
  i_d/1 -> Gain/1
  i_q/1 -> Gain1/1
  Product1/1 -> u_q_entk/1
  Product4/1 -> u_d_entk/1

== system gm_uz_pmsm_model_6LUT_pd_vnl/Current_Controller/Entkopplungen/dynamic_nonlinear_entkopplung1 ==
  i_d : Inport
  i_q : Inport  Port=2
  psi_d : Inport  Port=3
  psi_q : Inport  Port=4
  Ldq_LUT : Inport  Port=5
  Lqd_LUT : Inport  Port=6
  omega_m : Inport  Port=7
  Gain2 : Gain  Gain=polepair
  Product{,1..3} (4 alike) : Product
  Sum1 : Sum  Inputs=++|
  Sum6 : Sum  Inputs=++|
  u_d : Outport
  u_q : Outport  Port=2
  wires:
  psi_q/1 -> Product/1  "psi_q_LUT"
  Gain2/1 -> Product1/2, Product/2
  psi_d/1 -> Product1/1  "psi_d_LUT"
  omega_m/1 -> Gain2/1
  i_d/1 -> Product2/1
  Ldq_LUT/1 -> Product2/2
  Sum6/1 -> u_q/1
  Product1/1 -> Sum6/2
  Product/1 -> Sum1/2
  Sum1/1 -> u_d/1
  i_q/1 -> Product3/1
  Lqd_LUT/1 -> Product3/2
  Product3/1 -> Sum6/1
  Product2/1 -> Sum1/1

== system gm_uz_pmsm_model_6LUT_pd_vnl/Current_Controller/Entkopplungen/static_nonlinear_entkopplung ==
  psi_d : Inport
  psi_q : Inport  Port=2
  omega_m : Inport  Port=3
  Gain2 : Gain  Gain=polepair
  Product : Product
  Product1 : Product
  Scope : Scope  NumInputPorts=2
  u_d : Outport
  u_q : Outport  Port=2
  wires:
  psi_q/1 -> Product/1  "psi_q_LUT"
  Gain2/1 -> Product1/2, Product/2
  Product1/1 -> Scope/1, u_q/1
  Product/1 -> Scope/2, u_d/1
  psi_d/1 -> Product1/1  "psi_d_LUT"
  omega_m/1 -> Gain2/1

== system gm_uz_pmsm_model_6LUT_pd_vnl/uz_pmsm_model_6LUT_vnl/mechanical_system/integrator1 ==
  reset : Inport
  in : Inport  Port=2
  Delay1 : Delay  DelayLength=1  ExternalReset=Level
      settings: InputPortMap=u0,r5
  Gain : Gain  Gain=ts  OutDataTypeStr=double
  Sum3 : Sum  Inputs=|++  OutDataTypeStr=double
  outt : Outport
  wires:
  Delay1/1 -> outt/1, Sum3/2
  Sum3/1 -> Delay1/1
  reset/1 -> Delay1/2
  Gain/1 -> Sum3/1
  in/1 -> Gain/1

== system gm_uz_pmsm_model_6LUT_pd_vnl/uz_pmsm_model_6LUT_vnl/pmsm/Ldd_approx1 ==
  Id : Inport
  psiq_cross_s1_integrated : Inport  Port=2
  FittingParameters : Inport  Port=3
  Constant1 : Constant  SampleTime=ts
  Data Type Conversion1 : DataTypeConversion  OutDataTypeStr=double  RndMeth=Nearest  SaturateOnIntegerOverflow=off
  Data Type Conversion2 : DataTypeConversion  OutDataTypeStr=double  RndMeth=Nearest  SaturateOnIntegerOverflow=off
  Data Type Conversion6 : DataTypeConversion  OutDataTypeStr=single  RndMeth=Nearest  SaturateOnIntegerOverflow=off
  Data Type Conversion8 : DataTypeConversion  OutDataTypeStr=single  RndMeth=Nearest  SaturateOnIntegerOverflow=off
  Demux : Demux  Outputs=14
  Product : Product
  Product1 : Product  Inputs=3
  Product10 : Product  Inputs=3
  Product13 : Product  Inputs=*/
  Product14 : Product
  Product15 : Product
  Product16 : Product  Inputs=*/
  Product2 : Product  OutDataTypeStr=Inherit: Same as first input
  Product3 : Product  Inputs=3
  Sum{,1..2,7} (4 alike) : Sum  Inputs=|+-
  Tanh1 : Trigonometry  Operator=cosh
  Tanh4 : Trigonometry  Operator=cosh
  Terminator : Terminator
  Ldd : Outport
  wires:
  psiq_cross_s1_integrated/1 -> Product10/2
  Data Type Conversion8/1 -> Tanh1/1
  Data Type Conversion6/1 -> Tanh4/1
  Data Type Conversion2/1 -> Product13/2
  Data Type Conversion1/1 -> Product16/2
  Product15/1 -> Data Type Conversion1/1
  Product16/1 -> Product3/1
  Tanh1/1 -> Product15/1, Product15/2
  Constant1/1 -> Product13/1, Product16/1
  Tanh4/1 -> Product14/2, Product14/1
  Product14/1 -> Data Type Conversion2/1
  Demux/13 -> Product10/3  "F1G1"
  Demux/14 -> Terminator/1
  Sum7/1 -> Ldd/1  "psid_cross_s1"
  Product10/1 -> Sum7/2  "psid_cross"
  Sum2/1 -> Product10/1  "psid_cross_s1_abgeleitet"
  Product2/1 -> Data Type Conversion8/1
  Product3/1 -> Sum2/2  "psid_s1"
  Id/1 -> Sum/1, Sum1/1
  Demux/6 -> Sum1/2  "ad6"
  Demux/5 -> Product2/2, Product3/3  "ad5"
  Sum1/1 -> Product2/1
  Demux/4 -> Product3/2  "ad4"
  Product1/1 -> Sum2/1, Sum7/1  "psidself_abgeleitet"
  Product13/1 -> Product1/1
  Product/1 -> Data Type Conversion6/1
  Demux/2 -> Product/2, Product1/3  "ad2"
  Sum/1 -> Product/1
  Demux/3 -> Sum/2  "ad3"
  Demux/1 -> Product1/2  "ad1"
  FittingParameters/1 -> Demux/1

== system gm_uz_pmsm_model_6LUT_pd_vnl/uz_pmsm_model_6LUT_vnl/pmsm/Ldq ==
  psid_cross_s1 : Inport
  psiq_cross_s1 : Inport  Port=2
  FittingParameters : Inport  Port=3
  Demux : Demux  Outputs=14
  Gain : Gain  Gain=-1
  Product20 : Product  Inputs=3
  Terminator : Terminator
  psiq : Outport
  wires:
  psiq_cross_s1/1 -> Product20/2
  Demux/13 -> Product20/3
  Demux/14 -> Terminator/1
  Gain/1 -> psiq/1
  psid_cross_s1/1 -> Product20/1
  Product20/1 -> Gain/1  "psiq_cross"
  FittingParameters/1 -> Demux/1

== system gm_uz_pmsm_model_6LUT_pd_vnl/uz_pmsm_model_6LUT_vnl/pmsm/Lqd ==
  psid_cross_s1 : Inport
  psiq_cross_s1 : Inport  Port=2
  FittingParameters : Inport  Port=3
  Demux : Demux  Outputs=14
  Gain : Gain  Gain=-1
  Product20 : Product  Inputs=3
  Terminator : Terminator
  psiq : Outport
  wires:
  psiq_cross_s1/1 -> Product20/2
  Gain/1 -> psiq/1
  Demux/14 -> Product20/3
  psid_cross_s1/1 -> Product20/1
  Demux/13 -> Terminator/1
  Product20/1 -> Gain/1  "psiq_cross"
  FittingParameters/1 -> Demux/1

== system gm_uz_pmsm_model_6LUT_pd_vnl/uz_pmsm_model_6LUT_vnl/pmsm/Lqq_approx1 ==
  psid_cross_s1_integrated : Inport
  Iq : Inport  Port=2
  FittingParameters : Inport  Port=3
  Constant1 : Constant  SampleTime=ts
  Data Type Conversion2 : DataTypeConversion  OutDataTypeStr=double  RndMeth=Nearest  SaturateOnIntegerOverflow=off
  Data Type Conversion4 : DataTypeConversion  OutDataTypeStr=single  RndMeth=Nearest  SaturateOnIntegerOverflow=off
  Data Type Conversion5 : DataTypeConversion  OutDataTypeStr=single  RndMeth=Nearest  SaturateOnIntegerOverflow=off
  Data Type Conversion6 : DataTypeConversion  OutDataTypeStr=double  RndMeth=Nearest  SaturateOnIntegerOverflow=off
  Demux : Demux  Outputs=14
  Product : Product  OutDataTypeStr=Inherit: Same as first input
  Product1 : Product  Inputs=3
  Product13 : Product  Inputs=*/
  Product14 : Product
  Product15 : Product
  Product16 : Product  Inputs=*/
  Product2 : Product  OutDataTypeStr=Inherit: Same as first input
  Product20 : Product  Inputs=3
  Product3 : Product  Inputs=3
  Sum1 : Sum  Inputs=|++
  Sum10 : Sum  Inputs=|+-
  Sum2 : Sum  Inputs=|+-
  Sum4 : Sum  Inputs=|++
  Tanh1 : Trigonometry  Operator=cosh
  Tanh3 : Trigonometry  Operator=cosh
  Terminator : Terminator
  Lqq : Outport
  wires:
  psid_cross_s1_integrated/1 -> Product20/2
  Data Type Conversion6/1 -> Product13/2
  Data Type Conversion5/1 -> Tanh3/1
  Data Type Conversion4/1 -> Tanh1/1
  Data Type Conversion2/1 -> Product16/2
  Product3/1 -> Sum4/1  "psid_s1"
  Sum4/1 -> Sum2/2
  Sum1/1 -> Sum2/1, Sum10/1
  Product1/1 -> Sum1/1  "psidself_abgeleitet"
  Demux/7 -> Product1/2  "aq1"
  Demux/11 -> Product3/3, Product2/2  "aq5"
  Product/1 -> Data Type Conversion5/1
  Iq/1 -> Product/1, Product2/1
  Product2/1 -> Data Type Conversion4/1
  Demux/8 -> Product1/3, Product/2  "aq2"
  Demux/10 -> Product3/2  "aq4"
  Product14/1 -> Data Type Conversion6/1
  Product16/1 -> Product3/1
  Product13/1 -> Product1/1
  Sum2/1 -> Product20/1
  Tanh1/1 -> Product15/1, Product15/2
  Tanh3/1 -> Product14/2, Product14/1
  Constant1/1 -> Product13/1, Product16/1
  Demux/9 -> Sum1/2  "aq3"
  Product15/1 -> Data Type Conversion2/1
  Demux/13 -> Terminator/1
  Demux/14 -> Product20/3
  Sum10/1 -> Lqq/1  "Lqq"
  Product20/1 -> Sum10/2  "psiq_cross"
  Demux/12 -> Sum4/2  "aq6"
  FittingParameters/1 -> Demux/1

== system gm_uz_pmsm_model_6LUT_pd_vnl/uz_pmsm_model_6LUT_vnl/pmsm/Subsystem ==
  in : Inport
  reset : Inport  Port=2
  Delay1 : Delay  DelayLength=1  ExternalReset=Level
      settings: InputPortMap=u0,r5
  Gain7 : Gain  Gain=ts
  Sum5 : Sum  Inputs=|++
  outt : Outport
  wires:
  Gain7/1 -> Sum5/1  "u_d"
  Sum5/1 -> Delay1/1
  Delay1/1 -> Sum5/2, outt/1
  reset/1 -> Delay1/2
  in/1 -> Gain7/1

== system gm_uz_pmsm_model_6LUT_pd_vnl/uz_pmsm_model_6LUT_vnl/pmsm/Subsystem1 ==
  in : Inport
  reset : Inport  Port=2
  Delay1 : Delay  DelayLength=1  ExternalReset=Level
      settings: InputPortMap=u0,r5
  Gain7 : Gain  Gain=ts
  Sum5 : Sum  Inputs=|++
  outt : Outport
  wires:
  Gain7/1 -> Sum5/1  "u_d"
  Sum5/1 -> Delay1/1
  Delay1/1 -> Sum5/2, outt/1
  reset/1 -> Delay1/2
  in/1 -> Gain7/1

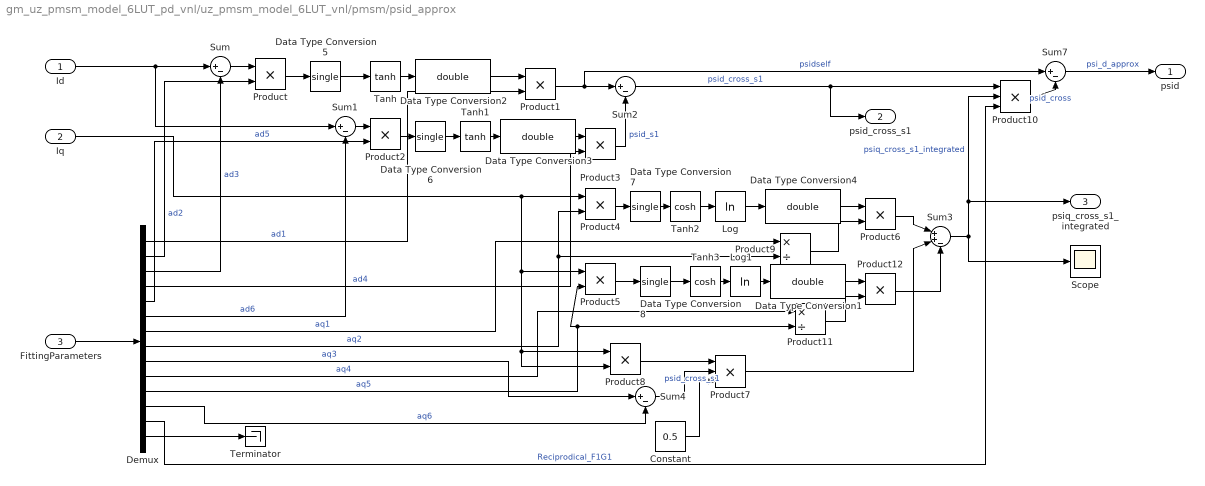
== system gm_uz_pmsm_model_6LUT_pd_vnl/uz_pmsm_model_6LUT_vnl/pmsm/psid_approx ==
  Id : Inport
  Iq : Inport  Port=2
  FittingParameters : Inport  Port=3
  Constant : Constant  Value=0.5  SampleTime=-1
  Data Type Conversion{1..4} (4 alike) : DataTypeConversion  OutDataTypeStr=double  RndMeth=Nearest  SaturateOnIntegerOverflow=off
  Data Type Conversion{5..8} (4 alike) : DataTypeConversion  OutDataTypeStr=single  RndMeth=Nearest  SaturateOnIntegerOverflow=off
  Demux : Demux  Outputs=14
  Log : Math  Operator=log  SignedPower=on
  Log1 : Math  Operator=log  SignedPower=on
  Product{,2,4..5} (4 alike) : Product  OutDataTypeStr=Inherit: Same as first input
  Product{1,3,6,8,12} (5 alike) : Product
  Product10 : Product  Inputs=3
  Product11 : Product  Inputs=*/
  Product7 : Product  Inputs=3
  Product9 : Product  Inputs=*/
  Scope : Scope
  Sum{,1..2,4,7} (5 alike) : Sum  Inputs=|+-
  Sum3 : Sum  Inputs=|++-
  Tanh : Trigonometry  Operator=tanh
  Tanh1 : Trigonometry  Operator=tanh
  Tanh2 : Trigonometry  Operator=cosh
  Tanh3 : Trigonometry  Operator=cosh
  Terminator : Terminator
  psid : Outport
  psid_cross_s1 : Outport  Port=2
  psiq_cross_s1_integrated : Outport  Port=3
  wires:
  Data Type Conversion8/1 -> Tanh3/1
  Product4/1 -> Data Type Conversion7/1
  Data Type Conversion7/1 -> Tanh2/1
  Data Type Conversion6/1 -> Tanh1/1
  Product2/1 -> Data Type Conversion6/1
  Data Type Conversion5/1 -> Tanh/1
  Data Type Conversion3/1 -> Product3/1
  Data Type Conversion2/1 -> Product1/1
  Data Type Conversion1/1 -> Product12/1
  Data Type Conversion4/1 -> Product6/1
  Demux/13 -> Product10/3  "Reciprodical_F1G1"
  Demux/14 -> Terminator/1
  Sum7/1 -> psid/1  "psi_d_approx"
  Product10/1 -> Sum7/2  "psid_cross"
  Demux/12 -> Sum4/2  "aq6"
  Demux/8 -> Product9/2, Product4/2  "aq2"
  Demux/11 -> Product11/2, Product5/2  "aq5"
  Demux/9 -> Sum4/1  "aq3"
  Demux/7 -> Product9/1  "aq1"
  Demux/10 -> Product11/1  "aq4"
  Sum3/1 -> Scope/1, psiq_cross_s1_integrated/1, Product10/2  "psiq_cross_s1_integrated"
  Constant/1 -> Product7/3
  Product12/1 -> Sum3/3
  Log1/1 -> Data Type Conversion1/1
  Product11/1 -> Product12/2
  Product6/1 -> Sum3/1
  Log/1 -> Data Type Conversion4/1
  Product9/1 -> Product6/2
  Product7/1 -> Sum3/2
  Product8/1 -> Product7/1
  Sum4/1 -> Product7/2  "psid_cross_s1"
  Product5/1 -> Data Type Conversion8/1
  Tanh3/1 -> Log1/1
  Tanh2/1 -> Log/1
  Sum2/1 -> Product10/1, psid_cross_s1/1  "psid_cross_s1"
  Iq/1 -> Product4/1, Product5/1, Product8/1, Product8/2
  Product3/1 -> Sum2/2  "psid_s1"
  Id/1 -> Sum/1, Sum1/1
  Tanh1/1 -> Data Type Conversion3/1
  Demux/6 -> Sum1/2  "ad6"
  Demux/5 -> Product2/2  "ad5"
  Sum1/1 -> Product2/1
  Demux/4 -> Product3/2  "ad4"
  Product1/1 -> Sum2/1, Sum7/1  "psidself"
  Tanh/1 -> Data Type Conversion2/1
  Product/1 -> Data Type Conversion5/1
  Demux/2 -> Product/2  "ad2"
  Sum/1 -> Product/1
  Demux/3 -> Sum/2  "ad3"
  Demux/1 -> Product1/2  "ad1"
  FittingParameters/1 -> Demux/1

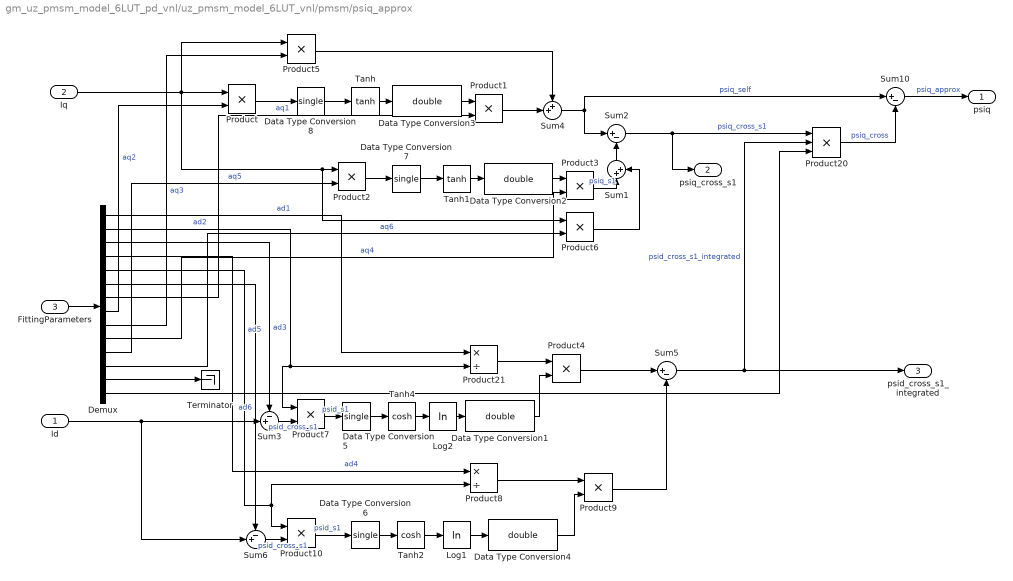
== system gm_uz_pmsm_model_6LUT_pd_vnl/uz_pmsm_model_6LUT_vnl/pmsm/psiq_approx ==
  Id : Inport
  Iq : Inport  Port=2
  FittingParameters : Inport  Port=3
  Data Type Conversion{1..4} (4 alike) : DataTypeConversion  OutDataTypeStr=double  RndMeth=Nearest  SaturateOnIntegerOverflow=off
  Data Type Conversion{5..8} (4 alike) : DataTypeConversion  OutDataTypeStr=single  RndMeth=Nearest  SaturateOnIntegerOverflow=off
  Demux : Demux  Outputs=14
  Log1 : Math  Operator=log  SignedPower=on
  Log2 : Math  Operator=log  SignedPower=on
  Product{,2,7,10} (4 alike) : Product  OutDataTypeStr=Inherit: Same as first input
  Product{1,3..6,9} (6 alike) : Product
  Product20 : Product  Inputs=3
  Product21 : Product  Inputs=*/
  Product8 : Product  Inputs=*/
  Sum1 : Sum  Inputs=|++
  Sum10 : Sum  Inputs=|+-
  Sum2 : Sum  Inputs=|+-
  Sum3 : Sum  Inputs=-+|
  Sum4 : Sum  Inputs=++|
  Sum5 : Sum  Inputs=|+-
  Sum6 : Sum  Inputs=-+|
  Tanh : Trigonometry  Operator=tanh
  Tanh1 : Trigonometry  Operator=tanh
  Tanh2 : Trigonometry  Operator=cosh
  Tanh4 : Trigonometry  Operator=cosh
  Terminator : Terminator
  psiq : Outport
  psiq_cross_s1 : Outport  Port=2
  psid_cross_s1_integrated : Outport  Port=3
  wires:
  Data Type Conversion8/1 -> Tanh/1
  Data Type Conversion7/1 -> Tanh1/1
  Data Type Conversion6/1 -> Tanh2/1
  Data Type Conversion5/1 -> Tanh4/1
  Data Type Conversion3/1 -> Product1/1
  Data Type Conversion2/1 -> Product3/1
  Data Type Conversion1/1 -> Product4/2
  Data Type Conversion4/1 -> Product9/2
  Demux/13 -> Terminator/1
  Demux/14 -> Product20/3
  Sum10/1 -> psiq/1  "psiq_approx"
  Product20/1 -> Sum10/2  "psiq_cross"
  Sum5/1 -> psid_cross_s1_integrated/1, Product20/2  "psid_cross_s1_integrated"
  Id/1 -> Sum3/2, Sum6/2
  Demux/6 -> Sum6/1  "ad6"
  Demux/5 -> Product10/1, Product8/2  "ad5"
  Demux/2 -> Product21/2, Product7/1  "ad2"
  Demux/4 -> Product8/1  "ad4"
  Demux/1 -> Product21/1  "ad1"
  Demux/3 -> Sum3/1  "ad3"
  Sum6/1 -> Product10/2  "psid_cross_s1"
  Log1/1 -> Data Type Conversion4/1
  Product8/1 -> Product9/1
  Tanh2/1 -> Log1/1
  Product10/1 -> Data Type Conversion6/1  "psid_s1"
  Product9/1 -> Sum5/2
  Product4/1 -> Sum5/1
  Product7/1 -> Data Type Conversion5/1  "psid_s1"
  Sum3/1 -> Product7/2  "psid_cross_s1"
  Product6/1 -> Sum1/2
  Product3/1 -> Sum1/1  "psiq_s1"
  Sum1/1 -> Sum2/2
  Sum4/1 -> Sum2/1, Sum10/1  "psiq_self"
  Product5/1 -> Sum4/1
  Product1/1 -> Sum4/2
  Product21/1 -> Product4/1
  Tanh4/1 -> Log2/1
  Log2/1 -> Data Type Conversion1/1
  Demux/9 -> Product5/2  "aq3"
  Iq/1 -> Product5/1, Product/1, Product6/1, Product2/1
  Tanh1/1 -> Data Type Conversion2/1
  Demux/7 -> Product1/2  "aq1"
  Tanh/1 -> Data Type Conversion3/1
  Demux/11 -> Product2/2  "aq5"
  Product/1 -> Data Type Conversion8/1
  Demux/8 -> Product/2  "aq2"
  Demux/12 -> Product6/2  "aq6"
  Product2/1 -> Data Type Conversion7/1
  Demux/10 -> Product3/2  "aq4"
  Sum2/1 -> psiq_cross_s1/1, Product20/1  "psiq_cross_s1"
  FittingParameters/1 -> Demux/1

== matlab function gm_uz_pmsm_model_6LUT_pd_vnl/Compare/Assert_outputs/RelErrCheck/RelativeErrorCheck  ==
  data: P input; y output; R input; ToleranceValue parameter double
% Check if the relative error of R with respect to P is below
% ToleranceValue
% P, R are floating-point
function y = relErrCheck(P,R, ToleranceValue)
    tol = ToleranceValue;
    sz = numel(P);
    assert(sz == numel(R), 'Inputs P and R have different sizes.');
    y = false(1, sz);

    for ii=1:sz
        if (isnan(P(ii)) || isnan(R(ii)))
            if (isnan(P(ii)) && isnan(R(ii)))
                y(ii) = true;
            end
        elseif (isinf(P(ii)) || isinf(R(ii)))
            y(ii) = (P(ii) == R(ii));
        elseif (P(ii) == 0)
            y(ii) = (R(ii) == 0);
        else
            absdiff = abs(P(ii) - R(ii));
            relerr = absdiff/abs(P(ii));
            y(ii) = (relerr <= tol);
        end
    end
end
